simulink model "DC_Motor_pt2"  (R2025a)
settings: Solver=VariableStepAuto  StartTime=0.0  StopTime=10.0  RelTol=1e-3
values from neighbouring files (symbols this model uses):
  A = [-R/L -Ke/L ; Kt/J 0]    [MotoreDC.m]    (also in MotoreDC_pt2.m = -beta./J)
  B = [1/L 0 ; 0 -1/J]    [MotoreDC.m]    (also in MotoreDC_pt2.m = 625000)
  beta = 4*J./ts    [MotoreDC_pt2.m]
  C = eye(2)    [MotoreDC.m]    (also in MotoreDC_pt2.m = 1)
  C_Rated = 2.0e-2    (= 0.02)    [MotoreDC_pt2.m]
  D = zeros(2)    [MotoreDC.m]    (also in MotoreDC_pt2.m = 0)
  J = 16e-7    (= 1.6e-06)    [MotoreDC.m]    (also in MotoreDC_pt2.m)
undefined symbols (not defined in the file or in its folder): C_Den_omega1, C_Den_omega2, C_Den_omega3, C_Den_omega4, C_Den_omega5, C_Den_omega6, C_Num_omega1, C_Num_omega2, C_Num_omega3, C_Num_omega4, C_Num_omega5, C_Num_omega6
settings Model: Creator=Mattia  LastModifiedBy=Mattia

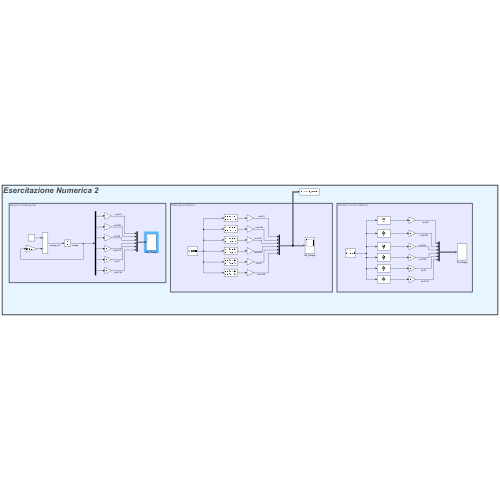
[thumbnail: Simulink's stored preview of the top-level diagram]
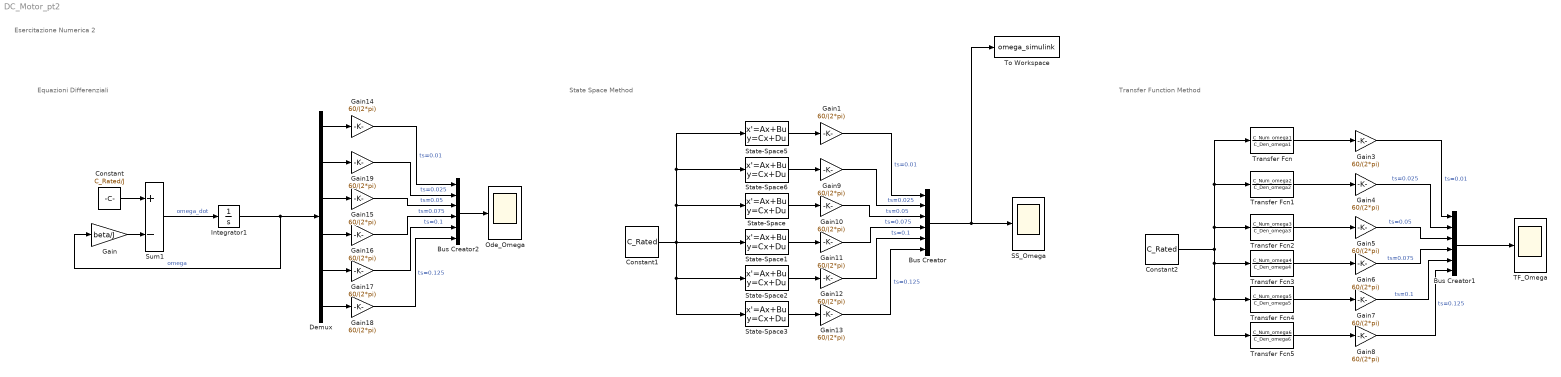
== system DC_Motor_pt2 ==
  note: Esercitazione Numerica 2
  note: Transfer Function Method
  note: State Space Method
  note: Equazioni Differenziali
  Bus Creator : BusCreator  Inputs=6
  Bus Creator1 : BusCreator  Inputs=6
  Bus Creator2 : BusCreator  Inputs=6
  Constant : Constant  Value=C_Rated/J
  Constant1 : Constant  Value=C_Rated
  Constant2 : Constant  Value=C_Rated
  Demux : Demux  Outputs=6
  Gain : Gain  Gain=beta/J
  Gain{1,3..19} (18 alike) : Gain  Gain=60/(2*pi)
  Integrator1 : Integrator
  Ode_Omega : Scope
      settings: ActiveDisplayYMinimum=-823.42205236614063  ActiveDisplayYMaximum=4376.8030436802137  DataLoggingVariableName=ScopeData3
  SS_Omega : Scope
      settings: ActiveDisplayYMinimum=-748.63653719996012  ActiveDisplayYMaximum=4175.5192713170554  DataLoggingVariableName=ScopeData2
  State-Space : StateSpace  A=A(3)  B=B  C=C  D=D  InitialCondition=0
  State-Space1 : StateSpace  A=A(4)  B=B  C=C  D=D  InitialCondition=0
  State-Space2 : StateSpace  A=A(5)  B=B  C=C  D=D  InitialCondition=0
  State-Space3 : StateSpace  A=A(6)  B=B  C=C  D=D  InitialCondition=0
  State-Space5 : StateSpace  A=A(1)  B=B  C=C  D=D  InitialCondition=0
  State-Space6 : StateSpace  A=A(2)  B=B  C=C  D=D  InitialCondition=0
  Sum1 : Sum  Inputs=+-
  TF_Omega : Scope
      settings: ActiveDisplayYMinimum=-634.16224265289065  ActiveDisplayYMaximum=4289.9935658641252
  To Workspace : ToWorkspace  VariableName=omega_simulink  SaveFormat=Timeseries  SampleTime=-1
  Transfer Fcn : TransferFcn  Numerator=C_Num_omega1  Denominator=C_Den_omega1
  Transfer Fcn1 : TransferFcn  Numerator=C_Num_omega2  Denominator=C_Den_omega2
  Transfer Fcn2 : TransferFcn  Numerator=C_Num_omega3  Denominator=C_Den_omega3
  Transfer Fcn3 : TransferFcn  Numerator=C_Num_omega4  Denominator=C_Den_omega4
  Transfer Fcn4 : TransferFcn  Numerator=C_Num_omega5  Denominator=C_Den_omega5
  Transfer Fcn5 : TransferFcn  Numerator=C_Num_omega6  Denominator=C_Den_omega6
  wires:
  Sum1/1 -> Integrator1/1  "omega_dot"
  Integrator1/1 -> Demux/1, Gain/1  "omega"
  Constant/1 -> Sum1/1
  Constant1/1 -> State-Space2/1, State-Space3/1, State-Space1/1, State-Space6/1, State-Space5/1, State-Space/1
  Gain/1 -> Sum1/2
  Constant2/1 -> Transfer Fcn/1, Transfer Fcn1/1, Transfer Fcn2/1, Transfer Fcn5/1, Transfer Fcn4/1, Transfer Fcn3/1
  Transfer Fcn/1 -> Gain3/1
  Transfer Fcn1/1 -> Gain4/1
  Transfer Fcn2/1 -> Gain5/1
  Transfer Fcn3/1 -> Gain6/1
  Transfer Fcn4/1 -> Gain7/1
  Transfer Fcn5/1 -> Gain8/1
  Gain8/1 -> Bus Creator1/6  "ts=0.125"
  Gain7/1 -> Bus Creator1/5  "ts=0.1"
  Gain6/1 -> Bus Creator1/4  "ts=0.075"
  Gain5/1 -> Bus Creator1/3  "ts=0.05"
  Gain4/1 -> Bus Creator1/2  "ts=0.025"
  Gain3/1 -> Bus Creator1/1  "ts=0.01"
  Gain1/1 -> Bus Creator/1  "ts=0.01"
  Gain11/1 -> Bus Creator/4  "ts=0.075"
  Gain9/1 -> Bus Creator/2  "ts=0.025"
  Gain12/1 -> Bus Creator/5  "ts=0.1"
  Gain10/1 -> Bus Creator/3  "ts=0.05"
  Gain13/1 -> Bus Creator/6  "ts=0.125"
  State-Space5/1 -> Gain1/1
  State-Space6/1 -> Gain9/1
  State-Space/1 -> Gain10/1
  State-Space1/1 -> Gain11/1
  State-Space2/1 -> Gain12/1
  State-Space3/1 -> Gain13/1
  Bus Creator/1 -> To Workspace/1, SS_Omega/1
  Bus Creator1/1 -> TF_Omega/1
  Gain14/1 -> Bus Creator2/1  "ts=0.01"
  Demux/2 -> Gain19/1
  Demux/3 -> Gain15/1
  Demux/6 -> Gain18/1
  Gain15/1 -> Bus Creator2/3  "ts=0.05"
  Demux/1 -> Gain14/1
  Gain17/1 -> Bus Creator2/5  "ts=0.1"
  Gain18/1 -> Bus Creator2/6  "ts=0.125"
  Demux/5 -> Gain17/1
  Demux/4 -> Gain16/1
  Gain16/1 -> Bus Creator2/4  "ts=0.075"
  Gain19/1 -> Bus Creator2/2  "ts=0.025"
  Bus Creator2/1 -> Ode_Omega/1
